simulink model "Car_boundary_testingDec_27_downsample_2012b"  (Simulink 8.0)
settings: Solver=ode5  StartTime=0.0  StopTime=inf  FixedStep=sample_time  RelTol=1e-3
InitFcn:
  | sample_time=0.005;%0.004;%0.0025;%0.02;
  | sample_time_Vicon = 0.005;
  | DeltaT = 0.02;
  | g = 9.81;
  | H0 = g%0.3165;
  | Kl = 1;
  | 
  | Q6_mass = 0.825;
  | 
  | Q6_Omega_r = 1.5; %for horizon ref
  | Q6_Zeta_r = 0.5; %for horizon ref
  | Q6_Omega_r_h = 2;%for vertical ref
  | Q6_Zeta_r_h = 1; %for vertical ref
  | 
  | 
  | Q6_Omega = 1.5; %for horizon control
  | Q6_Zeta = 0.5; %for horizon control
  | Q6_Omega_h= 2; %for vertical control
  | Q6_Zeta_h = 0.7; %for vertical control
  | 
  | 
  | Q6_acc_max = 5;%horizontal max acc
  | Q6_acc_max_h = 3;%horizontal max acc
  | 
  | omega_circle = 72*pi/180;
  | omega_h = 0.1;%Ascending speed
  | PI = pi;
  | Circle_R = 2.5;
  | MAX_Height = -2;
undefined symbols (not defined in the file): DiscIntNeverNeededParam
libraries: simulink x13, X330_Control x5, commsequence2 x5
(part 1 of 2)
settings Model: Creator=ttcl3  LastModifiedBy=eric
settings SolverCC: MaxConsecutiveMinStep=auto
settings DataIOCC: SignalLoggingSaveFormat=ModelDataLogs
settings DebuggingCC: MultiTaskRateTransMsg=warning  FcnCallInpInsideContextMsg=EnableAllAsWarning
settings SFSimCC: SimParseCustomCode=off
settings CodeAppCC: CustomSymbolStrType=$N$R$M_T
settings GRTTargetCC: CombineOutputUpdateFcns=off  GRTInterface=on

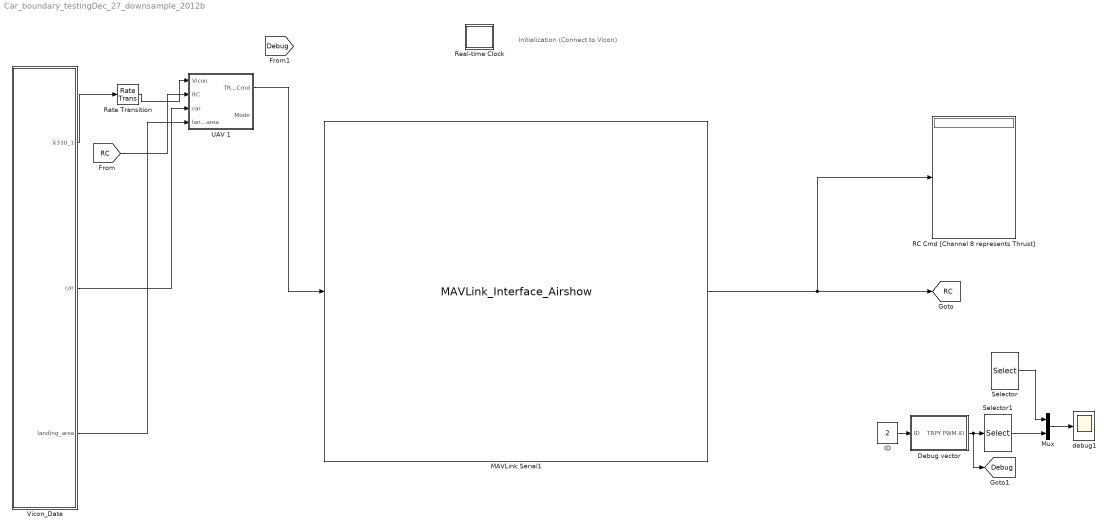
== system Car_boundary_testingDec_27_downsample_2012b ==
  note: Initialization
      | (Connect to Vicon)
  Debug vector : Subsystem
  ID : Constant  Value=2
  MAVLink Serial1 : S-Function  FunctionName=MAVLink_Interface_Airshow  Parameters=COM_Port,Baud_Rate,MSG_INPUT,MSG_OUTPUT  EnableBusSupport=off  mask{COM_Port='COM8', Baud_Rate=57600, ATTITUDE_OUT=off, RC_SCALED=on, Quads_1=on, Quads_2=off, Quads_3=off, Quads_4=off, Quads_5=off, Quads_6=off}
      mask prompts: COM_Port "COM Port"; Baud_Rate "Baud Rate"; ATTITUDE_OUT "DEBUG"; RC_SCALED "RC CHANNELS SCALED"; Quads_1 "1 Quad"; Quads_2 "2 Quad"; Quads_3 "3 Quad"; Quads_4 "4 Quad"; Quads_5 "5 Quad"; Quads_6 "6 Quad"
      mask init:
      | MSG_ID_NUM_INPUT = [ uint8(221) uint8(222) uint8(223) uint8(224) uint8(225) uint8(226)];
      | MSG_ID_NAME_INPUT = [Quads_1 Quads_2 Quads_3 Quads_4 Quads_5 Quads_6];
      | 
      | MSG_ID_NUM_OUTPUT = [uint8(34) uint8(30)];
      | MSG_ID_NAME_OUTPUT = [RC_SCALED ATTITUDE_OUT ];
      | 
      | idx_input = find(MSG_ID_NAME_INPUT);
      | MSG_INPUT = MSG_ID_NUM_INPUT(idx_input);
      | 
      | idx_output = find(MSG_ID_NAME_OUTPUT);
      | MSG_OUTPUT = MSG_ID_NUM_OUTPUT(idx_output);
      mask Display:
      | % Block image
      | image(imread('10-inch Quad Heat Map.png'));
      | 
      | %Label block
      | fprintf('MAVLink Serial\n%s\n%dbps', COM_Port,  Baud_Rate)
      | 
      | 
      | %Label input ports
      | 
      | in = 1;
      | if (Quads_1 == 1)
      |     port_label('input', in, 'Quads_1');
      |     in = in + 1;
      | end
      | 
      | if (Quads_2 == 1)
      |     port_label('input', in, 'Quads_2');
      |     in = in + 1;
      | end
      | 
      | if (Quads_3 == 1)
      |     port_label('input', in, 'Quads_3');
      |     in = in + 1;
      | end
      | 
      | if (Quads_4 == 1)
      |     port_label('input', in, 'Quads_4');
      |     in = in + 1;
      | end
      | 
      | if (Quads_5 == 1)
      |     port_label('input', in, 'Quads_5');
      |     in = in + 1;
      | end
      | 
      | 
      | if (Quads_6 == 1)
      |     port_label('input', in, 'Quads_6');
      |     in = in + 1;
      | end
      | %Label output ports
      | 
      | out = 1;
      | if (RC_SCALED == 1)
      |     port_label('output', out, 'RC CMD');
      |     out = out + 1;
      | end
      | 
      | if (ATTITUDE_OUT == 1)
      |     port_label('output', out, 'DEBUG');
      |     out = out + 1;
      | end
  Mux : Mux  Inputs=2
  RC Cmd [Channel 8 represents Thrust] : Display
  Rate Transition : RateTransition  OutPortSampleTime=0.02
  Real-time Clock : Subsystem  mask(Real-time Clock){sample_time=0.02, tolerance=1}
      mask prompts: sample_time "Synchronize with real-time every n seconds:"; tolerance "Real-time warning tolerance (seconds):"
      mask help: Real-time Synchronization Block
      mask Help: This block synchronizes simulation time with the PC real-time clock or UNIX system clock. The first dialog entry is the period at which the clock is checked to insure real-time synchronization. The second dialog entry is the number of seconds that the simulation time must be within real-time before a warning is printed.
      mask Display: plot(0,0,100,100,[40,60,60,54,54,64,69,76,82,77,81,83,83,81,78,74,70,64,57,49,41,35,32,30,30,31,34,40,47,47,40,40],[90,90,85,85,80,79,76,87,80,70,64,57,49,41,33,28,24,22,21,23,25,31,37,46,56,65,73,78,80,85,85,90],[69,53,53],[64,50,73])
  Selector : Selector  InputPortWidth=6  IndexOptions=Index vector (dialog)  Indices=[3]  OutputSizes=1
  Selector1 : Selector  InputPortWidth=6  IndexOptions=Index vector (dialog)  Indices=1  OutputSizes=1
  UAV 1 : Subsystem
  Vicon_Data : Subsystem
  debug1 : Scope
      settings: TimeRange=10  YMin=-1  YMax=1
  tag scope: Debug=global, RC=global
  wires:
  [RC] -> UAV 1/2(RC)
  Vicon_Data/1(X330_1) -> Rate Transition/1
  Rate Transition/1 -> UAV 1/1(Vicon)
  Mux/1 -> debug1/1
  Debug vector/1(TRPY PWM ID) -> Selector1/1, [Debug]
  ID/1 -> Debug vector/1(ID)
  Selector/1 -> Mux/1
  Selector1/1 -> Mux/2
  UAV 1/1(TRPY Cmd) -> MAVLink Serial1/1
  Vicon_Data/2(car) -> UAV 1/3(car)
  Vicon_Data/3(landing_area) -> UAV 1/4(landing_area)
  MAVLink Serial1/1 -> [RC], RC Cmd [Channel 8 represents Thrust]/1

== system Car_boundary_testingDec_27_downsample_2012b/Debug vector ==
  note: 6x1 vector (usec, XYZRPY)
  ID : Inport
  Mux1 : Mux  Inputs=6
  PWM : Constant  Value=0
  Pitch : Constant  Value=0
  Roll : Constant  Value=0
  Sine Wave : Sin  SampleTime=0
  Thrust : Constant  Value=0
  Yaw : Constant  Value=0
  TRPY PWM ID : Outport
  wires:
  Mux1/1 -> TRPY PWM ID/1
  Roll/1 -> Mux1/2
  Pitch/1 -> Mux1/3
  Yaw/1 -> Mux1/4
  PWM/1 -> Mux1/5
  ID/1 -> Mux1/6
  Sine Wave/1 -> Mux1/1

== system Car_boundary_testingDec_27_downsample_2012b/Real-time Clock ==
  Real-time Clock : S-Function  FunctionName=rtclock  Parameters=sample_time, tolerance  EnableBusSupport=off

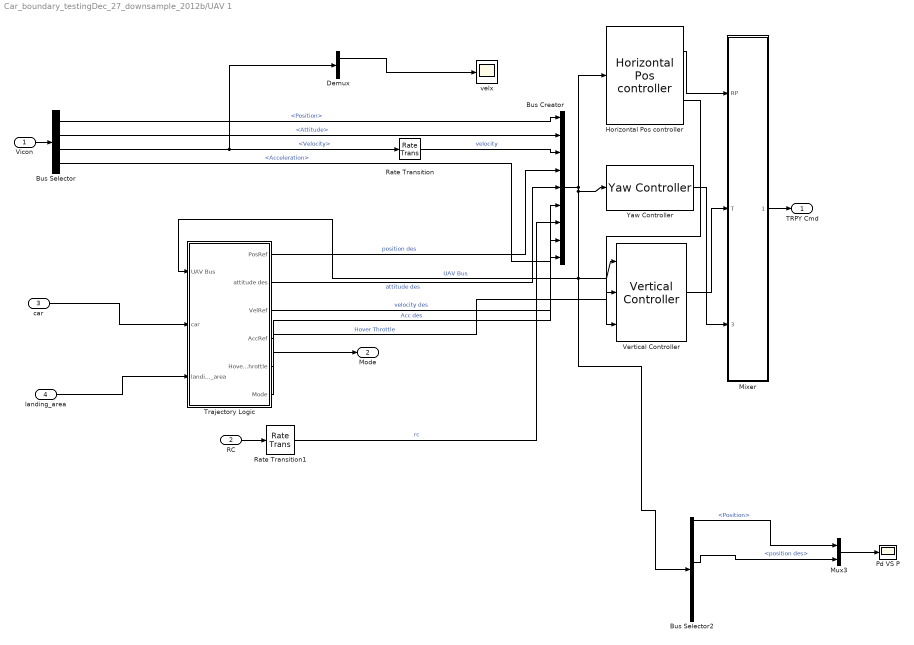
== system Car_boundary_testingDec_27_downsample_2012b/UAV 1 ==
  Vicon : Inport
  RC : Inport  Port=2
  car : Inport  Port=3
  landing_area : Inport  Port=4
  Bus Creator : BusCreator  Inputs=9
  Bus Selector : BusSelector  OutputSignals=Position,Attitude,Velocity,Acceleration
  Bus Selector2 : BusSelector  OutputSignals=Position,Attitude,velocity,position des,attitude des,velocity des,rc,Acc des
  Demux : Demux  Outputs=3
  Horizontal Pos controller : X330_Control/Horizontal Pos controller  Max_RP=60  Omega=Q6_Omega  PID_i=1  Zeta=Q6_Zeta
  Mixer : Subsystem
  Mux3 : Mux  Inputs=2
  Pd VS P : Scope
      settings: TimeRange=10  YMin=-3.5  YMax=3.5
  Rate Transition : RateTransition  OutPortSampleTime=0.02
  Rate Transition1 : RateTransition  OutPortSampleTime=0.02
  Trajectory Logic : Subsystem
  Vertical Controller : X330_Control/Vertical Controller  Omega_h=Q6_Omega_h  Zeta_h=Q6_Zeta_h  PID_I_h=1  mass=Q6_mass
  Yaw Controller : X330_Control/Yaw Controller
  velx : Scope
      settings: YMin=-4  YMax=4  SaveName=ScopeData8
  TRPY Cmd : Outport
  Mode : Outport  Port=2
  wires:
  Mux3/1 -> Pd VS P/1
  Bus Selector2/4 -> Mux3/2  "<position des>"
  Bus Selector2/1 -> Mux3/1  "<Position>"
  Horizontal Pos controller/2 -> Vertical Controller/3
  RC/1 -> Rate Transition1/1
  Trajectory Logic/6(Mode) -> Mode/1
  Trajectory Logic/4(AccRef) -> Bus Creator/9  "Acc des"
  Mixer/1(XYZ RPY) -> TRPY Cmd/1
  Vicon/1 -> Bus Selector/1
  Bus Selector/3 -> Demux/1, Rate Transition/1  "<Velocity>"
  Bus Selector/2 -> Bus Creator/2  "<Attitude>"
  Bus Selector/1 -> Bus Creator/1  "<Position>"
  Trajectory Logic/5(HoverThrottle) -> Vertical Controller/2  "Hover Throttle"
  Trajectory Logic/3(VelRef) -> Bus Creator/6  "velocity des"
  Trajectory Logic/2(attitude des) -> Bus Creator/5  "attitude des"
  Trajectory Logic/1(PosRef) -> Bus Creator/4  "position des"
  Bus Selector/4 -> Bus Creator/8  "<Acceleration>"
  Vertical Controller/1 -> Mixer/2(T)
  Yaw Controller/1 -> Mixer/3(Yaw rate)
  Bus Creator/1 -> Yaw Controller/1, Bus Selector2/1, Vertical Controller/1, Trajectory Logic/1(UAV Bus), Horizontal Pos controller/1  "UAV Bus"
  Rate Transition1/1 -> Bus Creator/7  "rc"
  Rate Transition/1 -> Bus Creator/3  "velocity"
  Horizontal Pos controller/1 -> Mixer/1(RP)
  car/1 -> Trajectory Logic/2(car)
  landing_area/1 -> Trajectory Logic/3(landing_area)
  Demux/1 -> velx/1

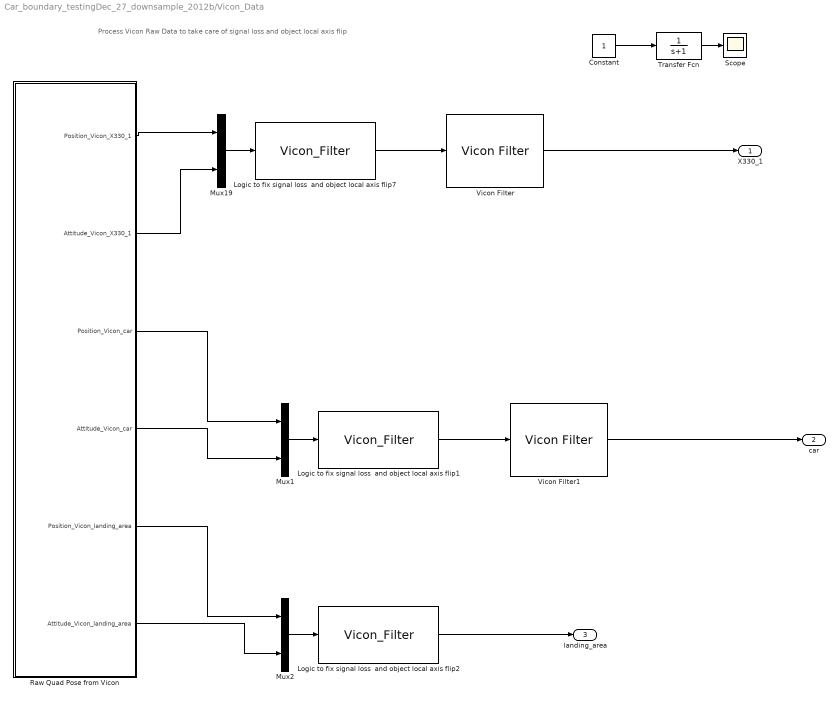
== system Car_boundary_testingDec_27_downsample_2012b/Vicon_Data ==
  note: Process Vicon Raw Data to take care of signal loss and object local axis flip
  Constant : Constant  SampleTime=5
  Logic to fix signal loss  and object local axis flip1 : M-S-Function  FunctionName=Vicon_Filter
  Logic to fix signal loss  and object local axis flip2 : M-S-Function  FunctionName=Vicon_Filter
  Logic to fix signal loss  and object local axis flip7 : M-S-Function  FunctionName=Vicon_Filter
  Mux1 : Mux  Inputs=2
  Mux19 : Mux  Inputs=2
  Mux2 : Mux  Inputs=2
  Raw Quad Pose from Vicon : Subsystem
  Scope : Scope
      settings: SaveName=ScopeData2
  Transfer Fcn : TransferFcn  Denominator=[1 1]
  Vicon Filter : X330_Control/Vicon Filter
  Vicon Filter1 : X330_Control/Vicon Filter
  X330_1 : Outport
  car : Outport  Port=2
  landing_area : Outport  Port=3
  wires:
  Mux19/1 -> Logic to fix signal loss  and object local axis flip7/1
  Raw Quad Pose from Vicon/1(Position_Vicon_X330_1) -> Mux19/1
  Raw Quad Pose from Vicon/2(Attitude_Vicon_X330_1) -> Mux19/2
  Logic to fix signal loss  and object local axis flip7/1 -> Vicon Filter/1
  Vicon Filter/1 -> X330_1/1
  Constant/1 -> Transfer Fcn/1
  Transfer Fcn/1 -> Scope/1
  Mux1/1 -> Logic to fix signal loss  and object local axis flip1/1
  Logic to fix signal loss  and object local axis flip1/1 -> Vicon Filter1/1
  Vicon Filter1/1 -> car/1
  Raw Quad Pose from Vicon/3(Position_Vicon_car) -> Mux1/1
  Raw Quad Pose from Vicon/4(Attitude_Vicon_car) -> Mux1/2
  Mux2/1 -> Logic to fix signal loss  and object local axis flip2/1
  Logic to fix signal loss  and object local axis flip2/1 -> landing_area/1
  Raw Quad Pose from Vicon/5(Position_Vicon_landing_area) -> Mux2/1
  Raw Quad Pose from Vicon/6(Attitude_Vicon_landing_area) -> Mux2/2

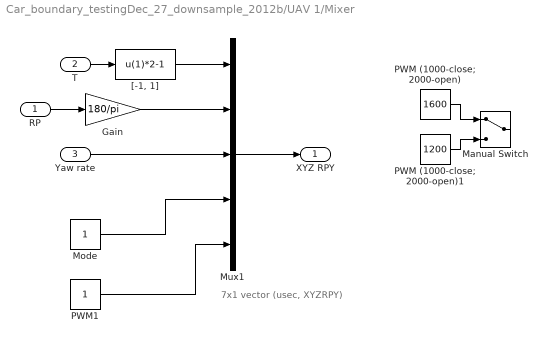
== system Car_boundary_testingDec_27_downsample_2012b/UAV 1/Mixer ==
  note: 7x1 vector (usec, XYZRPY)
  RP : Inport
  T : Inport  Port=2
  Yaw rate : Inport  Port=3
  Gain : Gain  Gain=180/pi
  Manual Switch : ManualSwitch
  Mode : Constant  SampleTime=0.02
  Mux1 : Mux  Inputs=5
  PWM (1000-close; 2000-open) : Constant  Value=1600  SampleTime=0.02
  PWM (1000-close; 2000-open)1 : Constant  Value=1200  SampleTime=0.02
  PWM1 : Constant  SampleTime=0.02
  "[-1, 1]" : Fcn  Expr=u(1)*2-1
  XYZ RPY : Outport
  wires:
  "[-1, 1]"/1 -> Mux1/1
  Gain/1 -> Mux1/2
  PWM (1000-close; 2000-open)1/1 -> Manual Switch/2
  PWM (1000-close; 2000-open)/1 -> Manual Switch/1
  Yaw rate/1 -> Mux1/3
  RP/1 -> Gain/1
  T/1 -> "[-1, 1]"/1
  Mux1/1 -> XYZ RPY/1
  Mode/1 -> Mux1/4
  PWM1/1 -> Mux1/5

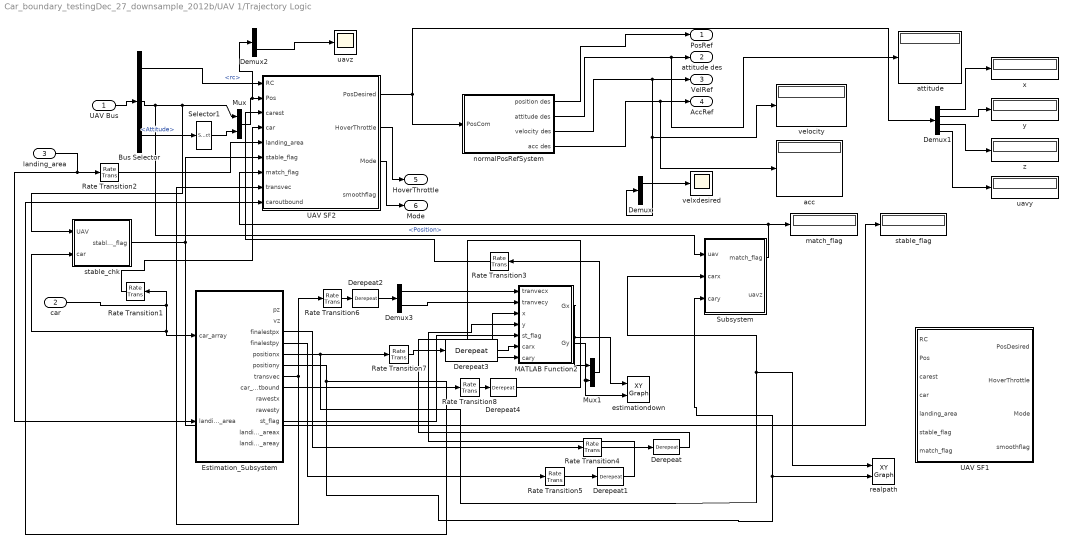
== system Car_boundary_testingDec_27_downsample_2012b/UAV 1/Trajectory Logic ==
  UAV Bus : Inport
  car : Inport  Port=2
  landing_area : Inport  Port=3
  Bus Selector : BusSelector  OutputSignals=rc,Position,Attitude
  Demux : Demux  Outputs=3
  Demux1 : Demux
  Demux2 : Demux  Outputs=3
  Demux3 : Demux  Outputs=2
  Derepeat{,1..4} (5 alike) : commsequence2/Derepeat  N=200  mode=Unused parameter value  InputProcessing=Columns as channels (frame based)  RateOptions=Allow multirate processing  ic=0
  Estimation_Subsystem : Subsystem
  MATLAB Function2 : MATLAB Function  TreatAsAtomicUnit=on
      settings: PermitHierarchicalResolution=ParametersOnly
  Mux : Mux  Inputs=2
  Mux1 : Mux  Inputs=2
  Rate Transition1 : RateTransition  OutPortSampleTime=0.02
  Rate Transition2 : RateTransition  OutPortSampleTime=0.02
  Rate Transition3 : RateTransition  OutPortSampleTime=1
  Rate Transition{4..8} (5 alike) : RateTransition  OutPortSampleTime=0.005
  Selector1 : Selector  InputPortWidth=3  IndexOptions=Index vector (dialog)  Indices=[3]  OutputSizes=1
  Subsystem : Subsystem
  UAV SF1 : Stateflow chart  TreatAsAtomicUnit=on
      settings: PermitHierarchicalResolution=ParametersOnly
  UAV SF2 : Stateflow chart  TreatAsAtomicUnit=on
      settings: PermitHierarchicalResolution=ParametersOnly
  acc : Display
  attitude : Display
  estimationdown : simulink/Sinks/XY Graph  xmin=-4  xmax=4  ymin=-4  ymax=4  st=-1
  match_flag : Display
  normalPosRefSystem : Subsystem  AncestorBlock=X330_Control/PosRefSystem  mask{Omega_r=Q6_Omega_r, Zeta_r=Q6_Zeta_r, Acc_Max=Q6_acc_max, Omega_h_r=Q6_Omega_r_h, Zeta_h_r=Q6_Zeta_r_h, Acc_h_Max=Q6_acc_max_h}
      mask prompts: Omega_r "Omega_r (P Gain= Omega_r^2)"; Zeta_r "Zeta_r (D = 2*Omega_r*Zeta_r)"
  realpath : simulink/Sinks/XY Graph  xmin=-4  xmax=4  ymin=-4  ymax=4  st=-1
  stable_chk : Subsystem
  stable_flag : Display
  uavy : Display
  uavz : Scope
      settings: YMin=-2.25  YMax=2.25  SaveName=ScopeData12
  velocity : Display
  velxdesired : Scope
      settings: YMin=-2.25  YMax=2.25  SaveName=ScopeData9
  x : Display
  y : Display
  z : Display
  PosRef : Outport
  attitude des : Outport  Port=2
  VelRef : Outport  Port=3
  AccRef : Outport  Port=4
  HoverThrottle : Outport  Port=5
  Mode : Outport  Port=6
  wires:
  Mux/1 -> Demux2/1, UAV SF2/2(Pos)
  Selector1/1 -> Mux/2
  Bus Selector/3 -> Selector1/1  "<Attitude>"
  Bus Selector/2 -> Mux/1, stable_chk/1(UAV), Subsystem/1(uav)  "<Position>"
  UAV Bus/1 -> Bus Selector/1
  UAV SF2/3(Mode) -> Mode/1
  UAV SF2/2(HoverThrottle) -> HoverThrottle/1
  Bus Selector/1 -> UAV SF2/1(RC)  "<rc>"
  car/1 -> Estimation_Subsystem/1(car_array), stable_chk/2(car), Rate Transition1/1
  Estimation_Subsystem/5(positionx) -> Rate Transition7/1, realpath/1, Subsystem/2(carx)
  Estimation_Subsystem/6(positiony) -> Subsystem/3(cary), realpath/2, Rate Transition8/1
  landing_area/1 -> Rate Transition2/1, Estimation_Subsystem/2(landing_area)
  stable_chk/1(stable_flag) -> UAV SF2/6(stable_flag), stable_flag/1
  Subsystem/1(match_flag) -> UAV SF2/7(match_flag), match_flag/1
  UAV SF2/1(PosDesired) -> Demux1/1, normalPosRefSystem/1(PosCom)
  normalPosRefSystem/3(velocity des) -> Demux/1, velocity/1, VelRef/1
  normalPosRefSystem/1(position des) -> PosRef/1
  normalPosRefSystem/4(acc des) -> acc/1, AccRef/1
  Demux1/1 -> x/1
  Demux1/2 -> y/1
  Demux1/3 -> z/1
  Demux1/4 -> uavy/1
  Estimation_Subsystem/7(transvec) -> Rate Transition6/1, UAV SF2/8(transvec)
  normalPosRefSystem/2(attitude des) -> attitude/1, attitude des/1
  Estimation_Subsystem/8(car_outbound) -> UAV SF2/9(caroutbound)
  Rate Transition2/1 -> UAV SF2/5(landing_area)
  Rate Transition1/1 -> UAV SF2/4(car)
  Demux/1 -> velxdesired/1
  Demux2/3 -> uavz/1
  Estimation_Subsystem/3(finalestpx) -> Rate Transition4/1
  Estimation_Subsystem/4(finalestpy) -> Rate Transition5/1
  Rate Transition4/1 -> Derepeat/1
  Rate Transition5/1 -> Derepeat1/1
  Rate Transition3/1 -> UAV SF2/3(carest)
  Estimation_Subsystem/11(st_flag) -> MATLAB Function2/5(st_flag)
  Derepeat/1 -> MATLAB Function2/3(x)
  Derepeat1/1 -> MATLAB Function2/4(y)
  MATLAB Function2/1(Gx) -> estimationdown/1, Mux1/1
  MATLAB Function2/2(Gy) -> estimationdown/2, Mux1/2
  Mux1/1 -> Rate Transition3/1
  Demux3/1 -> MATLAB Function2/1(tranvecx)
  Demux3/2 -> MATLAB Function2/2(tranvecy)
  Derepeat2/1 -> Demux3/1
  Rate Transition6/1 -> Derepeat2/1
  Derepeat3/1 -> MATLAB Function2/6(carx)
  Rate Transition8/1 -> Derepeat4/1
  Derepeat4/1 -> MATLAB Function2/7(cary)
  Rate Transition7/1 -> Derepeat3/1

== system Car_boundary_testingDec_27_downsample_2012b/Vicon_Data/Raw Quad Pose from Vicon ==
  Constant : Constant  SampleTime=sample_time
  Demux : Demux  Outputs=3
  Interpreted MATLAB Function : MATLABFcn  MATLABFcn=GetViconPose_car  OutputDimensions=18
  Process Vicon Raw Data-UAV : Subsystem
  Process Vicon Raw Data-car : Subsystem
  Process Vicon Raw Data-landing_area : Subsystem
  Position_Vicon_X330_1 : Outport
  Attitude_Vicon_X330_1 : Outport  Port=2
  Position_Vicon_car : Outport  Port=3
  Attitude_Vicon_car : Outport  Port=4
  Position_Vicon_landing_area : Outport  Port=5
  Attitude_Vicon_landing_area : Outport  Port=6
  wires:
  Interpreted MATLAB Function/1 -> Demux/1
  Process Vicon Raw Data-UAV/2(Attitude) -> Attitude_Vicon_X330_1/1
  Process Vicon Raw Data-UAV/1(Position) -> Position_Vicon_X330_1/1
  Demux/1 -> Process Vicon Raw Data-UAV/1(Vicon Raw)
  Constant/1 -> Interpreted MATLAB Function/1
  Process Vicon Raw Data-car/2(Attitude) -> Attitude_Vicon_car/1
  Process Vicon Raw Data-car/1(Position) -> Position_Vicon_car/1
  Demux/2 -> Process Vicon Raw Data-car/1(Vicon Raw)
  Process Vicon Raw Data-landing_area/2(Attitude) -> Attitude_Vicon_landing_area/1
  Process Vicon Raw Data-landing_area/1(Position) -> Position_Vicon_landing_area/1
  Demux/3 -> Process Vicon Raw Data-landing_area/1(Vicon Raw)

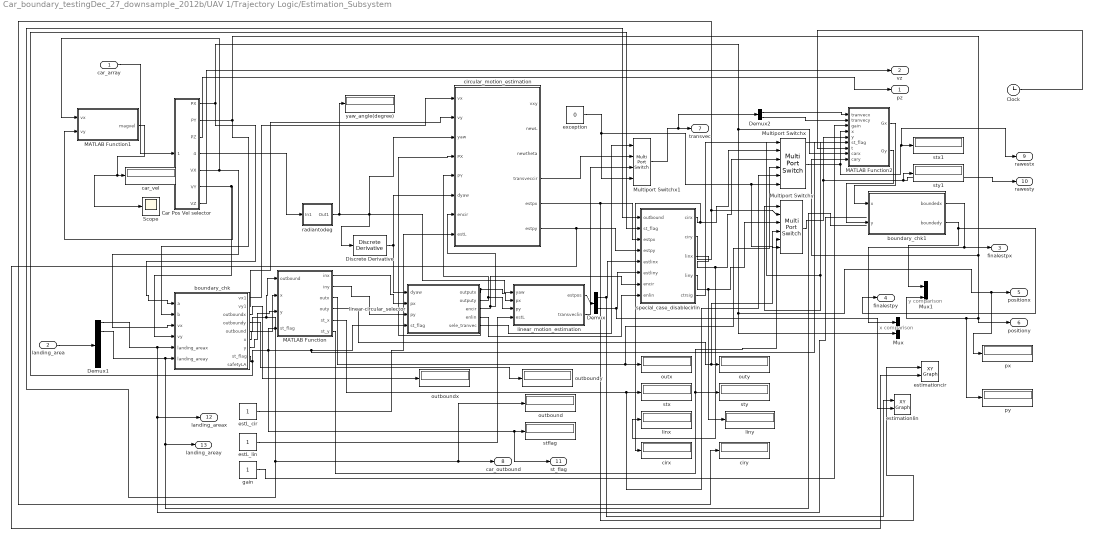
== system Car_boundary_testingDec_27_downsample_2012b/UAV 1/Trajectory Logic/Estimation_Subsystem ==
  note: y comparison
  note: x comparison
  car_array : Inport
  landing_area : Inport  Port=2
  Car Pos Vel selector : Subsystem
  Clock : Clock
  Demux : Demux  Outputs=2
  Demux1 : Demux  Outputs=6
  Demux2 : Demux  Outputs=2
  Discrete Derivative : simulink/Discrete/Discrete Derivative  gainval=1.0  ICPrevScaledInput=0.0  InputProcessing=Inherited  OutMin=[]  OutMax=[]  OutDataType=fixdt(1, 16)  OutScaling=2^-10  DoSatur=off
  MATLAB Function : MATLAB Function  TreatAsAtomicUnit=on
      settings: PermitHierarchicalResolution=ParametersOnly
  MATLAB Function1 : MATLAB Function  TreatAsAtomicUnit=on
      settings: PermitHierarchicalResolution=ParametersOnly
  MATLAB Function2 : MATLAB Function  TreatAsAtomicUnit=on
      settings: PermitHierarchicalResolution=ParametersOnly
  Multiport Switchx : MultiPortSwitch  Inputs=5
  Multiport Switchx1 : MultiPortSwitch
  Multiport Switchy : MultiPortSwitch  Inputs=5
  Mux : Mux  Inputs=2
  Mux1 : Mux  Inputs=2
  Scope : Scope
      settings: YMin=0  YMax=3.5  SaveName=ScopeData7
  boundary_chk : MATLAB Function  TreatAsAtomicUnit=on
      settings: PermitHierarchicalResolution=ParametersOnly
  boundary_chk1 : MATLAB Function  TreatAsAtomicUnit=on
      settings: PermitHierarchicalResolution=ParametersOnly
  car_vel : Display
  circular_motion_estimation : Subsystem
  cirx : Display
  ciry : Display
  estL_cir : Constant
  estL_lin : Constant
  estimationcir : simulink/Sinks/XY Graph  xmin=-4  xmax=4  ymin=-4  ymax=4  st=-1
  estimationlin : simulink/Sinks/XY Graph  xmin=-4  xmax=4  ymin=-4  ymax=4  st=-1
  exception : Constant  Value=0
  "gain " : Constant
  linear-circular_selector : MATLAB Function  TreatAsAtomicUnit=on
      settings: PermitHierarchicalResolution=ParametersOnly
  linear_motion_estimation : MATLAB Function  TreatAsAtomicUnit=on
      settings: PermitHierarchicalResolution=ParametersOnly
  linx : Display
  liny : Display
  outbound : Display
  outboundx : Display
  outboundy : Display
  outx : Display
  outy : Display
  px : Display
  py : Display
  radiantodeg : Subsystem
  special_case_disablecirlin : MATLAB Function  TreatAsAtomicUnit=on
      settings: PermitHierarchicalResolution=ParametersOnly
  stflag : Display
  stx : Display
  stx1 : Display
  sty : Display
  sty1 : Display
  yaw_angle(degree) : Display
  pz : Outport
  vz : Outport  Port=2
  finalestpx : Outport  Port=3
  finalestpy : Outport  Port=4
  positionx : Outport  Port=5
  positiony : Outport  Port=6
  transvec : Outport  Port=7
  car_outbound : Outport  Port=8
  rawestx : Outport  Port=9
  rawesty : Outport  Port=10
  st_flag : Outport  Port=11
  landing_areax : Outport  Port=12
  landing_areay : Outport  Port=13
  wires:
  Car Pos Vel selector/7(VZ) -> vz/1
  Car Pos Vel selector/3(PZ) -> pz/1
  Car Pos Vel selector/1("PX ") -> boundary_chk/1(a), MATLAB Function2/8(carx), Mux/2, px/1, positionx/1
  car_array/1 -> Car Pos Vel selector/1(car)
  Car Pos Vel selector/2(PY) -> boundary_chk/2(b), MATLAB Function2/9(cary), py/1, Mux1/2, positiony/1
  Car Pos Vel selector/4(yaw) -> radiantodeg/1(In1)
  Car Pos Vel selector/5(VX) -> MATLAB Function1/1(vx), boundary_chk/3(vx)
  Car Pos Vel selector/6(VY) -> MATLAB Function1/2(vy), boundary_chk/4(vy)
  radiantodeg/1(Out1) -> yaw_angle(degree)/1, Discrete Derivative/1, linear_motion_estimation/1(yaw), circular_motion_estimation/3(yaw)
  Discrete Derivative/1 -> circular_motion_estimation/6(dyaw), linear-circular_selector/1(dyaw)
  linear-circular_selector/1(outputx) -> circular_motion_estimation/4(PX), linear_motion_estimation/2(px)
  linear-circular_selector/3(encir) -> special_case_disablecirlin/7(encir), circular_motion_estimation/7(encir)
  linear-circular_selector/4(enlin) -> special_case_disablecirlin/8(enlin)
  linear_motion_estimation/1(estpos) -> Demux/1
  Demux/1 -> estimationlin/1, special_case_disablecirlin/5(estlinx)
  Demux/2 -> estimationlin/2, special_case_disablecirlin/6(estliny)
  linear-circular_selector/2(outputy) -> linear_motion_estimation/3(py), circular_motion_estimation/5(PY)
  boundary_chk/5(outbound) -> outbound/1, car_outbound/1, special_case_disablecirlin/1(outbound), MATLAB Function/1(outbound)
  boundary_chk/6(x) -> MATLAB Function/2(x)
  boundary_chk/7(y) -> MATLAB Function/3(y)
  boundary_chk/8(st_flag) -> MATLAB Function/4(st_flag), MATLAB Function2/6(st_flag), linear-circular_selector/4(st_flag), st_flag/1, stflag/1, special_case_disablecirlin/2(st_flag)
  MATLAB Function/1(inx) -> linear-circular_selector/2(px)
  MATLAB Function/2(iny) -> linear-circular_selector/3(py)
  MATLAB Function/4(outy) -> Multiport Switchy/4, outy/1
  MATLAB Function/5(st_x) -> Multiport Switchx/5, stx/1
  MATLAB Function/6(st_y) -> Multiport Switchy/5, sty/1
  estL_cir/1 -> circular_motion_estimation/8(estL)
  estL_lin/1 -> linear_motion_estimation/4(estL)
  boundary_chk/1(vx1) -> circular_motion_estimation/1(vx)
  boundary_chk/2(vy1) -> circular_motion_estimation/2(vy)
  circular_motion_estimation/4(transveccir) -> Multiport Switchx1/2
  linear_motion_estimation/2(transveclin) -> Multiport Switchx1/3
  Multiport Switchx1/1 -> Demux2/1, transvec/1
  landing_area/1 -> Demux1/1
  Demux1/1 -> landing_areax/1, boundary_chk/5(landing_areax)
  Demux1/2 -> landing_areay/1, boundary_chk/6(landing_areay)
  circular_motion_estimation/5(estpx) -> estimationcir/1, special_case_disablecirlin/3(estpx)
  circular_motion_estimation/6(estpy) -> estimationcir/2, special_case_disablecirlin/4(estpy)
  special_case_disablecirlin/1(cirx) -> cirx/1, Multiport Switchx/2
  special_case_disablecirlin/3(linx) -> linx/1, Multiport Switchx/3
  special_case_disablecirlin/2(ciry) -> Multiport Switchy/2, ciry/1
  special_case_disablecirlin/4(liny) -> Multiport Switchy/3, liny/1
  special_case_disablecirlin/5(ctrsig) -> Multiport Switchy/1, Multiport Switchx/1
  MATLAB Function/3(outx) -> Multiport Switchx/4, outx/1
  MATLAB Function1/1(magvel) -> Scope/1, car_vel/1
  linear-circular_selector/5(sele_tranvec) -> Multiport Switchx1/1
  Demux2/1 -> MATLAB Function2/1(tranvecx)
  Demux2/2 -> MATLAB Function2/2(tranvecy)
  "gain "/1 -> MATLAB Function2/3(gain)
  Multiport Switchx/1 -> rawestx/1, stx1/1, MATLAB Function2/4(x)
  Multiport Switchy/1 -> rawesty/1, sty1/1, MATLAB Function2/5(y)
  exception/1 -> Multiport Switchy/6, Multiport Switchx/6, Multiport Switchx1/4
  Clock/1 -> MATLAB Function2/7(t)
  boundary_chk1/1(boundedx) -> Mux/1, finalestpx/1
  boundary_chk1/2(boundedy) -> Mux1/1, finalestpy/1
  boundary_chk/3(outboundx) -> outboundx/1
  boundary_chk/4(outboundy) -> outboundy/1
  MATLAB Function2/1(Gx) -> boundary_chk1/1(x)
  MATLAB Function2/2(Gy) -> boundary_chk1/2(y)

== system Car_boundary_testingDec_27_downsample_2012b/UAV 1/Trajectory Logic/Subsystem ==
  uav : Inport
  carx : Inport  Port=2
  cary : Inport  Port=3
  Demux : Demux  Outputs=3
  Subtractx : Sum  Inputs=+-
  Subtracty : Sum  Inputs=+-
  UAVvscarx : Scope
      settings: YMin=-4  YMax=2.5  SaveName=ScopeData5
  UAVvscary : Scope
      settings: YMin=0.75  YMax=3.5  SaveName=ScopeData6
  match_chk : MATLAB Function  TreatAsAtomicUnit=on
      settings: PermitHierarchicalResolution=ParametersOnly
  match_flag : Outport
  uavz : Outport  Port=2
  wires:
  Demux/2 -> Subtracty/1
  Demux/1 -> Subtractx/1
  Subtractx/1 -> match_chk/1(vsx), UAVvscarx/1
  Subtracty/1 -> match_chk/2(vsy), UAVvscary/1
  uav/1 -> Demux/1
  carx/1 -> Subtractx/2
  cary/1 -> Subtracty/2
  match_chk/1(match_flag) -> match_flag/1
  Demux/3 -> uavz/1

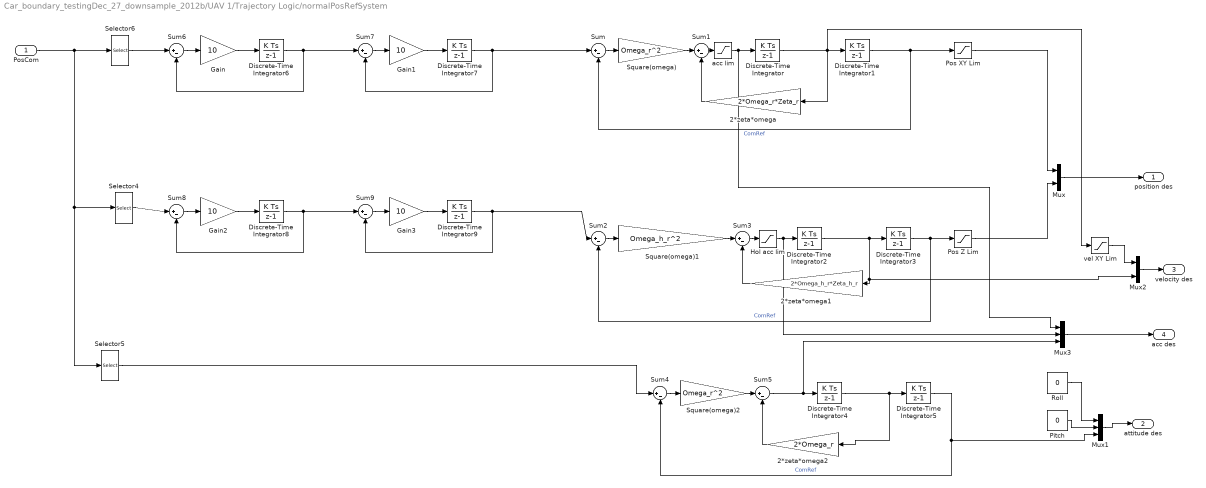
== system Car_boundary_testingDec_27_downsample_2012b/UAV 1/Trajectory Logic/normalPosRefSystem ==
  PosCom : Inport
  2*zeta*omega : Gain  Gain=2*Omega_r*Zeta_r
  2*zeta*omega1 : Gain  Gain=2*Omega_h_r*Zeta_h_r
  2*zeta*omega2 : Gain  Gain=2*Omega_r
  Discrete-Time Integrator{,1..9} (10 alike) : DiscreteIntegrator  SampleTime=-1  ICPrevOutput=DiscIntNeverNeededParam  ICPrevScaledInput=DiscIntNeverNeededParam
  Gain{,1..3} (4 alike) : Gain  Gain=10
  Hol acc lim : Saturate  UpperLimit=Acc_h_Max  LowerLimit=-Acc_h_Max
  Mux : Mux  Inputs=2
  Mux1 : Mux  Inputs=3
  Mux2 : Mux  Inputs=2
  Mux3 : Mux  Inputs=3
  Pitch : Constant  Value=0  SampleTime=0.02
  Pos XY Lim : Saturate  UpperLimit=3  LowerLimit=-3
  Pos Z Lim : Saturate  LowerLimit=-1.6
  Roll : Constant  Value=0  SampleTime=0.02
  Selector4 : Selector  InputPortWidth=4  IndexOptions=Index vector (dialog)  Indices=[3]  OutputSizes=1
  Selector5 : Selector  InputPortWidth=4  IndexOptions=Index vector (dialog)  Indices=[4]  OutputSizes=1
  Selector6 : Selector  InputPortWidth=4  IndexOptions=Index vector (dialog)  Indices=[1 2]  OutputSizes=1
  Square(omega) : Gain  Gain=Omega_r^2
  Square(omega)1 : Gain  Gain=Omega_h_r^2
  Square(omega)2 : Gain  Gain=Omega_r^2
  Sum{,1..9} (10 alike) : Sum  Inputs=|+-
  acc lim : Saturate  UpperLimit=Acc_Max  LowerLimit=-Acc_Max
  vel XY Lim : Saturate  UpperLimit=2.2  LowerLimit=-2.2
  position des : Outport
  attitude des : Outport  Port=2
  velocity des : Outport  Port=3
  acc des : Outport  Port=4
  wires:
  Pos Z Lim/1 -> Mux/2
  Pos XY Lim/1 -> Mux/1
  Sum9/1 -> Gain3/1
  Gain3/1 -> Discrete-Time Integrator9/1
  Discrete-Time Integrator9/1 -> Sum2/1, Sum9/2
  Sum8/1 -> Gain2/1
  Gain2/1 -> Discrete-Time Integrator8/1
  Discrete-Time Integrator8/1 -> Sum9/1, Sum8/2
  Selector4/1 -> Sum8/1
  Sum7/1 -> Gain1/1
  Gain1/1 -> Discrete-Time Integrator7/1
  Discrete-Time Integrator7/1 -> Sum/1, Sum7/2
  Sum6/1 -> Gain/1
  Gain/1 -> Discrete-Time Integrator6/1
  Discrete-Time Integrator6/1 -> Sum7/1, Sum6/2
  Selector6/1 -> Sum6/1
  Mux3/1 -> acc des/1
  Mux2/1 -> velocity des/1
  Mux1/1 -> attitude des/1
  Pitch/1 -> Mux1/2
  Roll/1 -> Mux1/1
  Mux/1 -> position des/1
  Discrete-Time Integrator1/1 -> Pos XY Lim/1, Sum/2  "ComRef"
  Selector5/1 -> Sum4/1
  2*zeta*omega2/1 -> Sum5/2
  Sum5/1 -> Mux3/3, Discrete-Time Integrator4/1
  Discrete-Time Integrator4/1 -> 2*zeta*omega2/1, Discrete-Time Integrator5/1
  Square(omega)2/1 -> Sum5/1
  Sum4/1 -> Square(omega)2/1
  Discrete-Time Integrator5/1 -> Mux1/3, Sum4/2  "ComRef"
  Hol acc lim/1 -> Mux3/2, Discrete-Time Integrator2/1
  2*zeta*omega1/1 -> Sum3/2
  Sum3/1 -> Hol acc lim/1
  Discrete-Time Integrator2/1 -> Mux2/2, 2*zeta*omega1/1, Discrete-Time Integrator3/1
  Square(omega)1/1 -> Sum3/1
  Sum2/1 -> Square(omega)1/1
  Discrete-Time Integrator3/1 -> Pos Z Lim/1, Sum2/2  "ComRef"
  acc lim/1 -> Mux3/1, Discrete-Time Integrator/1
  2*zeta*omega/1 -> Sum1/2
  Sum1/1 -> acc lim/1
  Discrete-Time Integrator/1 -> 2*zeta*omega/1, vel XY Lim/1, Discrete-Time Integrator1/1
  Square(omega)/1 -> Sum1/1
  Sum/1 -> Square(omega)/1
  PosCom/1 -> Selector6/1, Selector5/1, Selector4/1
  vel XY Lim/1 -> Mux2/1

== system Car_boundary_testingDec_27_downsample_2012b/UAV 1/Trajectory Logic/stable_chk ==
  UAV : Inport
  car : Inport  Port=2
  Demux1 : Demux  Outputs=2
  Demux2 : Demux  Outputs=2
  Selector : Selector  InputPortWidth=3  IndexOptions=Index vector (dialog)  Indices=[1 2]  OutputSizes=1
  Selector2 : Selector  InputPortWidth=12  IndexOptions=Index vector (dialog)  Indices=[1 2]  OutputSizes=1
  stablize_checking : MATLAB Function  TreatAsAtomicUnit=on
      settings: PermitHierarchicalResolution=ParametersOnly
  stable_flag : Outport
  wires:
  Selector/1 -> Demux1/1
  Demux1/1 -> stablize_checking/1(posx)
  Demux1/2 -> stablize_checking/2(posy)
  Selector2/1 -> Demux2/1
  Demux2/1 -> stablize_checking/3(carx)
  Demux2/2 -> stablize_checking/4(cary)
  UAV/1 -> Selector/1
  car/1 -> Selector2/1
  stablize_checking/1(stable_flag) -> stable_flag/1

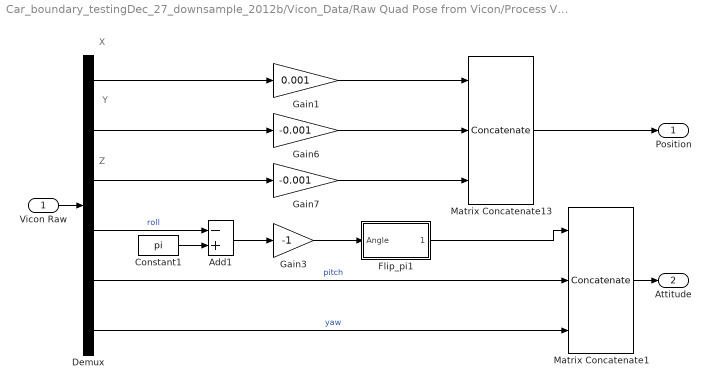
== system Car_boundary_testingDec_27_downsample_2012b/Vicon_Data/Raw Quad Pose from Vicon/Process Vicon Raw Data-UAV ==
  note: X
  note: Y
  note: Z
  Vicon Raw : Inport
  Add1 : Sum  Inputs=-+
  Constant1 : Constant  Value=pi  OutDataTypeStr=double
  Demux : Demux  Outputs=6
  Flip_pi1 : Subsystem  mask(Flip -pi to pi){}
      mask help: Flips the inputs into the range -pi to pi
      mask Help: Flips the inputs into the range -pi to pi
      mask Display: disp('Flip_pi')
  Gain1 : Gain  Gain=0.001
  Gain3 : Gain  Gain=-1
  Gain6 : Gain  Gain=-0.001
  Gain7 : Gain  Gain=-0.001
  Matrix Concatenate1 : Concatenate  NumInputs=3  Mode=Multidimensional array
  Matrix Concatenate13 : Concatenate  NumInputs=3  Mode=Multidimensional array
  Position : Outport
  Attitude : Outport  Port=2
  wires:
  Constant1/1 -> Add1/2
  Demux/6 -> Matrix Concatenate1/3  "yaw"
  Gain1/1 -> Matrix Concatenate13/1
  Demux/1 -> Gain1/1
  Demux/2 -> Gain6/1
  Demux/3 -> Gain7/1
  Demux/4 -> Add1/1  "roll"
  Gain6/1 -> Matrix Concatenate13/2
  Gain7/1 -> Matrix Concatenate13/3
  Add1/1 -> Gain3/1
  Gain3/1 -> Flip_pi1/1(Angle)
  Demux/5 -> Matrix Concatenate1/2  "pitch"
  Flip_pi1/1(Angle_Flip) -> Matrix Concatenate1/1
  Matrix Concatenate13/1 -> Position/1
  Vicon Raw/1 -> Demux/1
  Matrix Concatenate1/1 -> Attitude/1

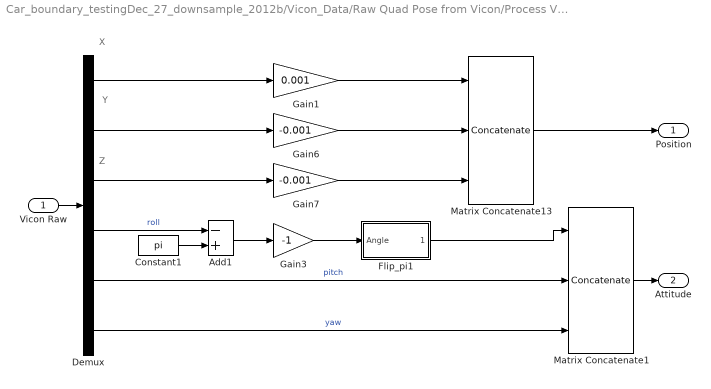
== system Car_boundary_testingDec_27_downsample_2012b/Vicon_Data/Raw Quad Pose from Vicon/Process Vicon Raw Data-car ==
  note: X
  note: Y
  note: Z
  Vicon Raw : Inport
  Add1 : Sum  Inputs=-+
  Constant1 : Constant  Value=pi  OutDataTypeStr=double
  Demux : Demux  Outputs=6
  Flip_pi1 : Subsystem  mask(Flip -pi to pi){}
      mask help: Flips the inputs into the range -pi to pi
      mask Help: Flips the inputs into the range -pi to pi
      mask Display: disp('Flip_pi')
  Gain1 : Gain  Gain=0.001
  Gain3 : Gain  Gain=-1
  Gain6 : Gain  Gain=-0.001
  Gain7 : Gain  Gain=-0.001
  Matrix Concatenate1 : Concatenate  NumInputs=3  Mode=Multidimensional array
  Matrix Concatenate13 : Concatenate  NumInputs=3  Mode=Multidimensional array
  Position : Outport
  Attitude : Outport  Port=2
  wires:
  Constant1/1 -> Add1/2
  Demux/6 -> Matrix Concatenate1/3  "yaw"
  Gain1/1 -> Matrix Concatenate13/1
  Demux/1 -> Gain1/1
  Demux/2 -> Gain6/1
  Demux/3 -> Gain7/1
  Demux/4 -> Add1/1  "roll"
  Gain6/1 -> Matrix Concatenate13/2
  Gain7/1 -> Matrix Concatenate13/3
  Add1/1 -> Gain3/1
  Gain3/1 -> Flip_pi1/1(Angle)
  Demux/5 -> Matrix Concatenate1/2  "pitch"
  Flip_pi1/1(Angle_Flip) -> Matrix Concatenate1/1
  Matrix Concatenate13/1 -> Position/1
  Vicon Raw/1 -> Demux/1
  Matrix Concatenate1/1 -> Attitude/1

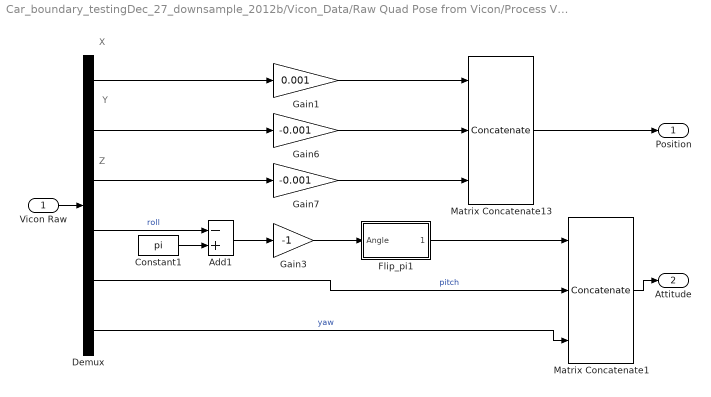
== system Car_boundary_testingDec_27_downsample_2012b/Vicon_Data/Raw Quad Pose from Vicon/Process Vicon Raw Data-landing_area ==
  note: X
  note: Y
  note: Z
  Vicon Raw : Inport
  Add1 : Sum  Inputs=-+
  Constant1 : Constant  Value=pi  OutDataTypeStr=double
  Demux : Demux  Outputs=6
  Flip_pi1 : Subsystem  mask(Flip -pi to pi){}
      mask help: Flips the inputs into the range -pi to pi
      mask Help: Flips the inputs into the range -pi to pi
      mask Display: disp('Flip_pi')
  Gain1 : Gain  Gain=0.001
  Gain3 : Gain  Gain=-1
  Gain6 : Gain  Gain=-0.001
  Gain7 : Gain  Gain=-0.001
  Matrix Concatenate1 : Concatenate  NumInputs=3  Mode=Multidimensional array
  Matrix Concatenate13 : Concatenate  NumInputs=3  Mode=Multidimensional array
  Position : Outport
  Attitude : Outport  Port=2
  wires:
  Constant1/1 -> Add1/2
  Demux/6 -> Matrix Concatenate1/3  "yaw"
  Gain1/1 -> Matrix Concatenate13/1
  Demux/1 -> Gain1/1
  Demux/2 -> Gain6/1
  Demux/3 -> Gain7/1
  Demux/4 -> Add1/1  "roll"
  Gain6/1 -> Matrix Concatenate13/2
  Gain7/1 -> Matrix Concatenate13/3
  Add1/1 -> Gain3/1
  Gain3/1 -> Flip_pi1/1(Angle)
  Demux/5 -> Matrix Concatenate1/2  "pitch"
  Flip_pi1/1(Angle_Flip) -> Matrix Concatenate1/1
  Matrix Concatenate13/1 -> Position/1
  Vicon Raw/1 -> Demux/1
  Matrix Concatenate1/1 -> Attitude/1

== system Car_boundary_testingDec_27_downsample_2012b/UAV 1/Trajectory Logic/Estimation_Subsystem/Car Pos Vel selector ==
  car : Inport
  Demux : Demux  Outputs=12
  "PX " : Outport
  PY : Outport  Port=2
  PZ : Outport  Port=3
  yaw : Outport  Port=4
  VX : Outport  Port=5
  VY : Outport  Port=6
  VZ : Outport  Port=7
  wires:
  car/1 -> Demux/1
  Demux/1 -> "PX "/1
  Demux/2 -> PY/1
  Demux/3 -> PZ/1
  Demux/6 -> yaw/1
  Demux/7 -> VX/1
  Demux/8 -> VY/1
  Demux/9 -> VZ/1

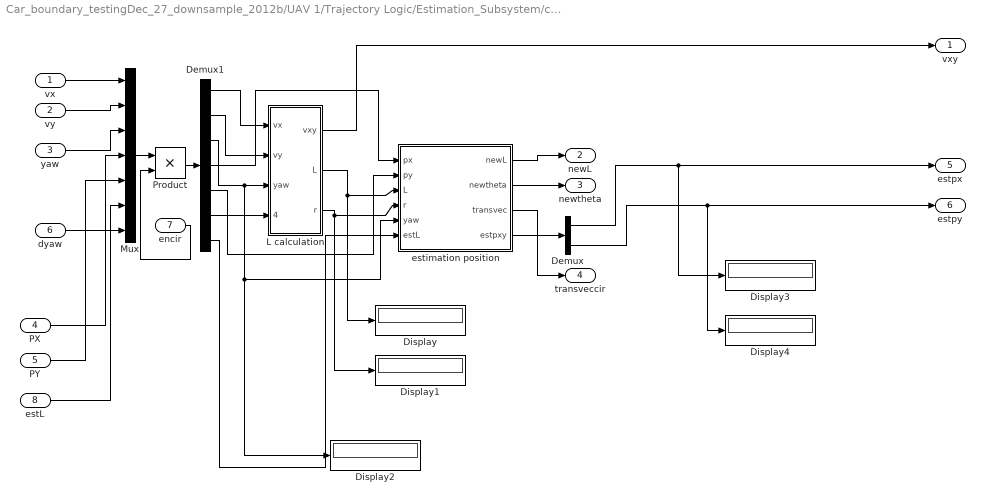
== system Car_boundary_testingDec_27_downsample_2012b/UAV 1/Trajectory Logic/Estimation_Subsystem/circular_motion_estimation ==
  vx : Inport
  vy : Inport  Port=2
  yaw : Inport  Port=3
  PX : Inport  Port=4
  PY : Inport  Port=5
  dyaw : Inport  Port=6
  encir : Inport  Port=7
  estL : Inport  Port=8
  Demux : Demux  Outputs=2
  Demux1 : Demux  Outputs=7
  Display{,1..4} (5 alike) : Display
  L calculation : Subsystem
  Mux : Mux  Inputs=7
  Product : Product
  estimation position : MATLAB Function  TreatAsAtomicUnit=on
      settings: PermitHierarchicalResolution=ParametersOnly
  vxy : Outport
  newL : Outport  Port=2
  newtheta : Outport  Port=3
  transveccir : Outport  Port=4
  estpx : Outport  Port=5
  estpy : Outport  Port=6
  wires:
  Demux/2 -> Display4/1, estpy/1
  L calculation/1(vxy) -> vxy/1
  estimation position/2(newtheta) -> newtheta/1
  estimation position/1(newL) -> newL/1
  estimation position/3(transvec) -> transveccir/1
  estimation position/4(estpxy) -> Demux/1
  vx/1 -> Mux/1
  vy/1 -> Mux/2
  yaw/1 -> Mux/3
  PX/1 -> Mux/4
  dyaw/1 -> Mux/6
  Mux/1 -> Product/1
  Product/1 -> Demux1/1
  encir/1 -> Product/2
  Demux1/1 -> L calculation/1(vx)
  Demux1/2 -> L calculation/2(vy)
  Demux1/3 -> Display2/1, estimation position/5(yaw), L calculation/3(yaw)
  Demux1/6 -> L calculation/4(dyaw)
  PY/1 -> Mux/5
  Demux/1 -> Display3/1, estpx/1
  L calculation/2(L) -> estimation position/3(L), Display/1
  L calculation/3("r ") -> estimation position/4(r), Display1/1
  Demux1/4 -> estimation position/1(px)
  Demux1/5 -> estimation position/2(py)
  estL/1 -> Mux/7
  Demux1/7 -> estimation position/6(estL)

== system Car_boundary_testingDec_27_downsample_2012b/UAV 1/Trajectory Logic/Estimation_Subsystem/radiantodeg ==
  In1 : Inport
  Constant : Constant  Value=180
  Constant1 : Constant  Value=pi
  Divide : Product  Inputs=*/
  Product : Product
  Out1 : Outport
  wires:
  Product/1 -> Out1/1
  Constant/1 -> Product/2
  Divide/1 -> Product/1
  In1/1 -> Divide/1
  Constant1/1 -> Divide/2

== system Car_boundary_testingDec_27_downsample_2012b/Vicon_Data/Raw Quad Pose from Vicon/Process Vicon Raw Data-UAV/Flip_pi1 ==
  Angle : Inport
  Add : Sum  Inputs=-+
  Compare To Constant1 : simulink/Logic and Bit Operations/Compare To Constant  relop=>  const=pi  OutDataTypeStr=uint8  ZeroCross=off
  Constant : Constant  Value=2*pi
  Data Type Duplicate : DataTypeDuplicate
  Flip_0_to_2pi : Subsystem  mask(Flip zero to 2pi){}
      mask help: Flips the inputs into the range zero to +2pi
      mask Help: Flips the inputs into the range zero to +2pi
      mask Display: disp('Flip_0_2pi')
  Switch : Switch  Criteria=u2 ~= 0
  Angle_Flip : Outport
  wires:
  Switch/1 -> Data Type Duplicate/1, Angle_Flip/1
  Add/1 -> Switch/1
  Constant/1 -> Add/1
  Compare To Constant1/1 -> Switch/2
  Flip_0_to_2pi/1(Angle_Flip) -> Add/2, Compare To Constant1/1, Switch/3
  Angle/1 -> Data Type Duplicate/2, Flip_0_to_2pi/1(Angle)

== system Car_boundary_testingDec_27_downsample_2012b/Vicon_Data/Raw Quad Pose from Vicon/Process Vicon Raw Data-car/Flip_pi1 ==
  Angle : Inport
  Add : Sum  Inputs=-+
  Compare To Constant1 : simulink/Logic and Bit Operations/Compare To Constant  relop=>  const=pi  OutDataTypeStr=uint8  ZeroCross=off
  Constant : Constant  Value=2*pi
  Data Type Duplicate : DataTypeDuplicate
  Flip_0_to_2pi : Subsystem  mask(Flip zero to 2pi){}
      mask help: Flips the inputs into the range zero to +2pi
      mask Help: Flips the inputs into the range zero to +2pi
      mask Display: disp('Flip_0_2pi')
  Switch : Switch  Criteria=u2 ~= 0
  Angle_Flip : Outport
  wires:
  Switch/1 -> Data Type Duplicate/1, Angle_Flip/1
  Add/1 -> Switch/1
  Constant/1 -> Add/1
  Compare To Constant1/1 -> Switch/2
  Flip_0_to_2pi/1(Angle_Flip) -> Add/2, Compare To Constant1/1, Switch/3
  Angle/1 -> Data Type Duplicate/2, Flip_0_to_2pi/1(Angle)

== system Car_boundary_testingDec_27_downsample_2012b/Vicon_Data/Raw Quad Pose from Vicon/Process Vicon Raw Data-landing_area/Flip_pi1 ==
  Angle : Inport
  Add : Sum  Inputs=-+
  Compare To Constant1 : simulink/Logic and Bit Operations/Compare To Constant  relop=>  const=pi  OutDataTypeStr=uint8  ZeroCross=off
  Constant : Constant  Value=2*pi
  Data Type Duplicate : DataTypeDuplicate
  Flip_0_to_2pi : Subsystem  mask(Flip zero to 2pi){}
      mask help: Flips the inputs into the range zero to +2pi
      mask Help: Flips the inputs into the range zero to +2pi
      mask Display: disp('Flip_0_2pi')
  Switch : Switch  Criteria=u2 ~= 0
  Angle_Flip : Outport
  wires:
  Switch/1 -> Data Type Duplicate/1, Angle_Flip/1
  Add/1 -> Switch/1
  Constant/1 -> Add/1
  Compare To Constant1/1 -> Switch/2
  Flip_0_to_2pi/1(Angle_Flip) -> Add/2, Compare To Constant1/1, Switch/3
  Angle/1 -> Data Type Duplicate/2, Flip_0_to_2pi/1(Angle)

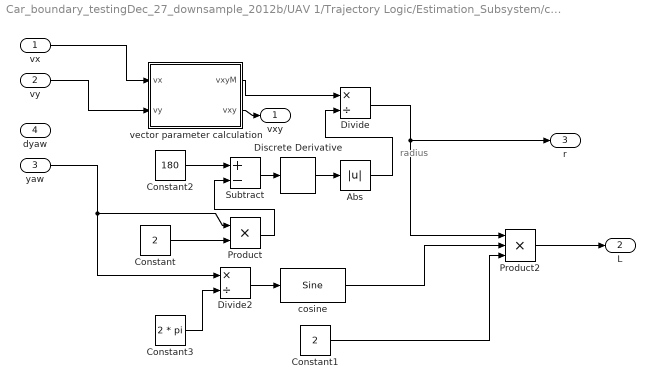
== system Car_boundary_testingDec_27_downsample_2012b/UAV 1/Trajectory Logic/Estimation_Subsystem/circular_motion_estimation/L calculation ==
  note: radius
  vx : Inport
  vy : Inport  Port=2
  yaw : Inport  Port=3
  dyaw : Inport  Port=4
  Abs : Abs
  Constant : Constant  Value=2
  Constant1 : Constant  Value=2
  Constant2 : Constant  Value=180
  Constant3 : Constant  Value=2 * pi
  Discrete Derivative : simulink/Discrete/Discrete Derivative  gainval=1.0  ICPrevScaledInput=0.0  InputProcessing=Inherited  OutMin=[]  OutMax=[]  OutDataType=fixdt(1, 16)  OutScaling=2^-10  DoSatur=off
  Divide : Product  Inputs=*/
  Divide2 : Product  Inputs=*/
  Product : Product
  Product2 : Product  Inputs=3
  Subtract : Sum  Inputs=+-
  cosine : simulink/Lookup Tables/Sine  Formula=cos(2*pi*u)  NumDataPoints=(2^5)+1  OutputWordLength=16
  vector parameter calculation : MATLAB Function  TreatAsAtomicUnit=on
      settings: PermitHierarchicalResolution=ParametersOnly
  vxy : Outport
  L : Outport  Port=2
  "r " : Outport  Port=3
  wires:
  vy/1 -> vector parameter calculation/2(vy)
  yaw/1 -> Product/1, Divide2/1
  Divide2/1 -> cosine/1
  Constant3/1 -> Divide2/2
  vector parameter calculation/1(vxyM) -> Divide/1
  Constant/1 -> Product/2
  vx/1 -> vector parameter calculation/1(vx)
  vector parameter calculation/2(vxy) -> vxy/1
  Abs/1 -> Divide/2
  cosine/1 -> Product2/2
  Product2/1 -> L/1
  Constant1/1 -> Product2/3
  Divide/1 -> "r "/1, Product2/1
  Constant2/1 -> Subtract/1
  Product/1 -> Subtract/2
  Subtract/1 -> Discrete Derivative/1
  Discrete Derivative/1 -> Abs/1

== system Car_boundary_testingDec_27_downsample_2012b/Vicon_Data/Raw Quad Pose from Vicon/Process Vicon Raw Data-UAV/Flip_pi1/Flip_0_to_2pi ==
  Angle : Inport
  Add : Sum
  Compare To Constant1 : simulink/Logic and Bit Operations/Compare To Constant  relop=<  const=0  OutDataTypeStr=uint8  ZeroCross=off
  Constant : Constant  Value=2*pi
  Data Type Duplicate : DataTypeDuplicate
  Flip_2pi : Subsystem  mask(Flip -2pi to 2pi){}
      mask help: Flips the inputs into the range -2pi to +2pi
      mask Help: Flips the inputs into the range -2pi to +2pi
      mask Display: disp('Flip_2pi')
  Switch : Switch  Criteria=u2 ~= 0
  Angle_Flip : Outport
  wires:
  Switch/1 -> Data Type Duplicate/1, Angle_Flip/1
  Angle/1 -> Data Type Duplicate/2, Flip_2pi/1(Angle)
  Add/1 -> Switch/1
  Constant/1 -> Add/1
  Compare To Constant1/1 -> Switch/2
  Flip_2pi/1(Angle_Flip) -> Switch/3, Add/2, Compare To Constant1/1

== system Car_boundary_testingDec_27_downsample_2012b/Vicon_Data/Raw Quad Pose from Vicon/Process Vicon Raw Data-car/Flip_pi1/Flip_0_to_2pi ==
  Angle : Inport
  Add : Sum
  Compare To Constant1 : simulink/Logic and Bit Operations/Compare To Constant  relop=<  const=0  OutDataTypeStr=uint8  ZeroCross=off
  Constant : Constant  Value=2*pi
  Data Type Duplicate : DataTypeDuplicate
  Flip_2pi : Subsystem  mask(Flip -2pi to 2pi){}
      mask help: Flips the inputs into the range -2pi to +2pi
      mask Help: Flips the inputs into the range -2pi to +2pi
      mask Display: disp('Flip_2pi')
  Switch : Switch  Criteria=u2 ~= 0
  Angle_Flip : Outport
  wires:
  Switch/1 -> Data Type Duplicate/1, Angle_Flip/1
  Angle/1 -> Data Type Duplicate/2, Flip_2pi/1(Angle)
  Add/1 -> Switch/1
  Constant/1 -> Add/1
  Compare To Constant1/1 -> Switch/2
  Flip_2pi/1(Angle_Flip) -> Switch/3, Add/2, Compare To Constant1/1

== system Car_boundary_testingDec_27_downsample_2012b/Vicon_Data/Raw Quad Pose from Vicon/Process Vicon Raw Data-landing_area/Flip_pi1/Flip_0_to_2pi ==
  Angle : Inport
  Add : Sum
  Compare To Constant1 : simulink/Logic and Bit Operations/Compare To Constant  relop=<  const=0  OutDataTypeStr=uint8  ZeroCross=off
  Constant : Constant  Value=2*pi
  Data Type Duplicate : DataTypeDuplicate
  Flip_2pi : Subsystem  mask(Flip -2pi to 2pi){}
      mask help: Flips the inputs into the range -2pi to +2pi
      mask Help: Flips the inputs into the range -2pi to +2pi
      mask Display: disp('Flip_2pi')
  Switch : Switch  Criteria=u2 ~= 0
  Angle_Flip : Outport
  wires:
  Switch/1 -> Data Type Duplicate/1, Angle_Flip/1
  Angle/1 -> Data Type Duplicate/2, Flip_2pi/1(Angle)
  Add/1 -> Switch/1
  Constant/1 -> Add/1
  Compare To Constant1/1 -> Switch/2
  Flip_2pi/1(Angle_Flip) -> Switch/3, Add/2, Compare To Constant1/1

== system Car_boundary_testingDec_27_downsample_2012b/Vicon_Data/Raw Quad Pose from Vicon/Process Vicon Raw Data-UAV/Flip_pi1/Flip_0_to_2pi/Flip_2pi ==
  Angle : Inport
  Bias : Bias  Bias=-2*pi
  Constant : Constant  Value=2*pi
  Data Type Duplicate : DataTypeDuplicate
  Modulo : Math  Operator=mod  SaturateOnIntegerOverflow=on
  Sign1 : Signum
  Switch : Switch
  Angle_Flip : Outport
  wires:
  Switch/1 -> Data Type Duplicate/2, Angle_Flip/1
  Bias/1 -> Switch/3
  Sign1/1 -> Switch/2
  Modulo/1 -> Switch/1, Bias/1
  Constant/1 -> Modulo/2
  Angle/1 -> Data Type Duplicate/1, Sign1/1, Modulo/1

== system Car_boundary_testingDec_27_downsample_2012b/Vicon_Data/Raw Quad Pose from Vicon/Process Vicon Raw Data-car/Flip_pi1/Flip_0_to_2pi/Flip_2pi ==
  Angle : Inport
  Bias : Bias  Bias=-2*pi
  Constant : Constant  Value=2*pi
  Data Type Duplicate : DataTypeDuplicate
  Modulo : Math  Operator=mod  SaturateOnIntegerOverflow=on
  Sign1 : Signum
  Switch : Switch
  Angle_Flip : Outport
  wires:
  Switch/1 -> Data Type Duplicate/2, Angle_Flip/1
  Bias/1 -> Switch/3
  Sign1/1 -> Switch/2
  Modulo/1 -> Switch/1, Bias/1
  Constant/1 -> Modulo/2
  Angle/1 -> Data Type Duplicate/1, Sign1/1, Modulo/1

== system Car_boundary_testingDec_27_downsample_2012b/Vicon_Data/Raw Quad Pose from Vicon/Process Vicon Raw Data-landing_area/Flip_pi1/Flip_0_to_2pi/Flip_2pi ==
  Angle : Inport
  Bias : Bias  Bias=-2*pi
  Constant : Constant  Value=2*pi
  Data Type Duplicate : DataTypeDuplicate
  Modulo : Math  Operator=mod  SaturateOnIntegerOverflow=on
  Sign1 : Signum
  Switch : Switch
  Angle_Flip : Outport
  wires:
  Switch/1 -> Data Type Duplicate/2, Angle_Flip/1
  Bias/1 -> Switch/3
  Sign1/1 -> Switch/2
  Modulo/1 -> Switch/1, Bias/1
  Constant/1 -> Modulo/2
  Angle/1 -> Data Type Duplicate/1, Sign1/1, Modulo/1

== matlab function UAV 1/Trajectory Logic/Estimation_Subsystem/circular_motion_estimation/estimation position ==
  data: px input double; py input double; newL output double; L input double; r input double; newtheta output double; yaw input double; transvec output double; estpxy output double; estL input double
function [newL, newtheta,transvec,estpxy]  = fcn(px,py,L,r,yaw,estL)
%#codegen
double angleOmega;%angle between new translation vector and orginal vx
 
if(r == 0)
    newL = 0;
    newtheta = 0;
else
if(L>=0)
    if(r<0.25)
        r = 0.25;
    end
newL = estL;
   if(estL > 2*r)
        estL = 2*r;
   end
   newtheta = acos(estL / (2 * r)) / pi * 180;
   
else
    newL = 0;
    newtheta = 0;
end
end
pxy = [px py];
angleOmega = 90 - newtheta + yaw;
transvec = [estL * cos(angleOmega) estL * sin(angleOmega)];
estpxy = pxy + transvec;

== matlab function UAV 1/Trajectory Logic/Estimation_Subsystem/circular_motion_estimation/L calculation/vector parameter calculation ==
  data: vxyM output double; vxy output double; vx input double; vy input double
function [vxyM,vxy] = fcn(vx,vy)
%#codegen
%magnitude M



vxyM = sqrt((vx)^2 + (vy)^2);
%resultant vector vxy

vxy = [vx vy];

== matlab function UAV 1/Trajectory Logic/Estimation_Subsystem/boundary_chk ==
  data: vx1 output double; vy1 output double; outboundx output double; outboundy output double; outbound output double; x output double; a input double; y output double; b input double; vx input double; vy input double; st_flag output double; landing_areax input double; landing_areay input double; safetyLA output double
function [vx1,vy1,outboundx,outboundy,outbound,x,y,st_flag,safetyLA] = fcn(a,b,vx,vy,landing_areax,landing_areay)
%#codegen

% define the boundry of a and b

vx1 = vx;
vy1 = vy;
if (a < -3)  
    x = -3;
    outboundx = 1;
elseif (a > 3)
    x = 3;
    outboundx = 1;
else
    x = a;
    outboundx = 0;
end

if (b < -3)
    y = -3;
    outboundy = 1;
elseif (b > 3)
      y = 3;
      outboundy = 1;
else
    y = b;
    outboundy = 0;
end

if(a > (landing_areax-1.45) && b >(landing_areay-1.45))
    safetyLA = 1;
%    x = landing_areax -1.45;
%    y = landing_areay - 1.45;
else
    safetyLA = 0;
end

if(outboundx == 1 || outboundy == 1)
    outbound = 1;
else
    outbound =0;
    
end

   

if (vx > -0.1 && vx < 0.1)
    vx1 = 0;
end
if(vy > -0.1 && vy < 0.1)
    vy1 = 0;
end
if(vx1 == 0 && vy1 == 0)
    st_flag = 1;
else 
    st_flag = 0;
end

== matlab function UAV 1/Trajectory Logic/Estimation_Subsystem/MATLAB Function ==
  data: outbound input double; x input double; y input double; st_flag input double; inx output double; iny output double; outx output double; outy output double; st_x output double; st_y output double
function [inx, iny, outx, outy, st_x, st_y] = fcn(outbound, x, y, st_flag)
%#codegen
if(outbound == 1)
    inx = 0;
    iny = 0;
    st_x = 0;
    st_y = 0;
    outx = x;
    outy = y;
else
    if(st_flag == 1)
        st_x = x;
        st_y = y;
        inx = 0;
        iny = 0;
        outx = 0;
        outy = 0;
    else
        inx = x;
        iny = y;
        st_x = 0;
        st_y = 0;
        outx = 0;
        outy = 0;
    end
end

== matlab function UAV 1/Trajectory Logic/Estimation_Subsystem/linear-circular_selector ==
  data: outputx output double; outputy output double; dyaw input double; encir output double; px input double; py input double; enlin output double; st_flag input double; sele_tranvec output double
function [outputx,outputy,encir,enlin,sele_tranvec] = fcn(dyaw,px,py,st_flag)
%#codegen

% select circular or linear estimation in the next sequence
if(st_flag == 0)
if(dyaw>-0.349 && dyaw < 0.349) %define yaw angle in 5 degree as linear motion
    dyaw = 0;
end
if(dyaw == 0)
    enlin = 1;
    encir = 0;
    sele_tranvec = 2;
else
    enlin = 0;
    encir = 1;
    sele_tranvec = 1;
   
end
    
else
    enlin = 0;
    encir = 0;
   sele_tranvec = 3;
end
outputx = px;
    outputy = py;

== matlab function UAV 1/Trajectory Logic/Estimation_Subsystem/linear_motion_estimation ==
  data: yaw input double; px input double; py input double; estpos output double; estL input double; transveclin output double
function [estpos,transveclin]  = fcn(yaw,px,py,estL)
%#codegen

%estimate linear motion

pxy = [px py];
transveclin = [estL * cos(yaw) estL * sin(yaw)];
estpos = pxy + transveclin;
